simulink model "dynamic_bicycle"  (R2019a)
settings: Solver=VariableStepAuto  StartTime=0.0  StopTime=20  RelTol=1e-3
values from neighbouring files (symbols this model uses):
  cornering_stiffness_front = 10000    [config_dynamic_bicycle.m]
  cornering_stiffness_rear = 10000    [config_dynamic_bicycle.m]
  init_states = [0,0,0,0,0,0]    [config_dynamic_bicycle.m]
  length_front = 1    [config_dynamic_bicycle.m]
  length_rear = 1    [config_dynamic_bicycle.m]
  mass = 200    [config_dynamic_bicycle.m]
  yaw_inertia = 50    [config_dynamic_bicycle.m]
libraries: simulink x2, simulink_extras x1
settings Model: Creator=jacoboffersen  LastModifiedBy=jacoboffersen

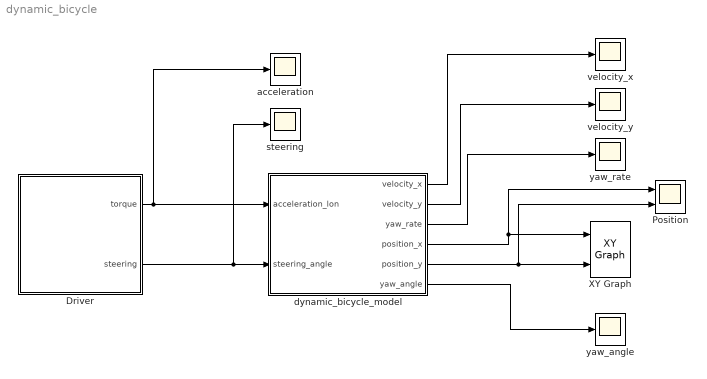
== system dynamic_bicycle ==
  Driver : Subsystem
  Position : Scope  NumInputPorts=2
  XY Graph : simulink/Sinks/XY Graph  xmin=-200  xmax=200  ymin=-200  ymax=200  st=-1
  acceleration : Scope
  "dynamic_bicycle_model " : Subsystem
  steering : Scope
  velocity_x : Scope
  velocity_y : Scope
  yaw_angle : Scope
  yaw_rate : Scope
  wires:
  Driver/2(steering) -> steering/1, "dynamic_bicycle_model "/2(steering_angle)
  Driver/1(torque) -> acceleration/1, "dynamic_bicycle_model "/1(acceleration_lon)
  "dynamic_bicycle_model "/4(position_x) -> Position/1, XY Graph/1
  "dynamic_bicycle_model "/5(position_y) -> Position/2, XY Graph/2
  "dynamic_bicycle_model "/6(yaw_angle) -> yaw_angle/1
  "dynamic_bicycle_model "/3(yaw_rate) -> yaw_rate/1
  "dynamic_bicycle_model "/2(velocity_y) -> velocity_y/1
  "dynamic_bicycle_model "/1(velocity_x) -> velocity_x/1

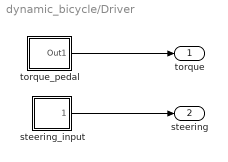
== system dynamic_bicycle/Driver ==
  steering_input : Subsystem
  torque_pedal : Subsystem
  torque : Outport
  steering : Outport  Port=2
  wires:
  torque_pedal/1(Out1) -> torque/1
  steering_input/1(Out1) -> steering/1

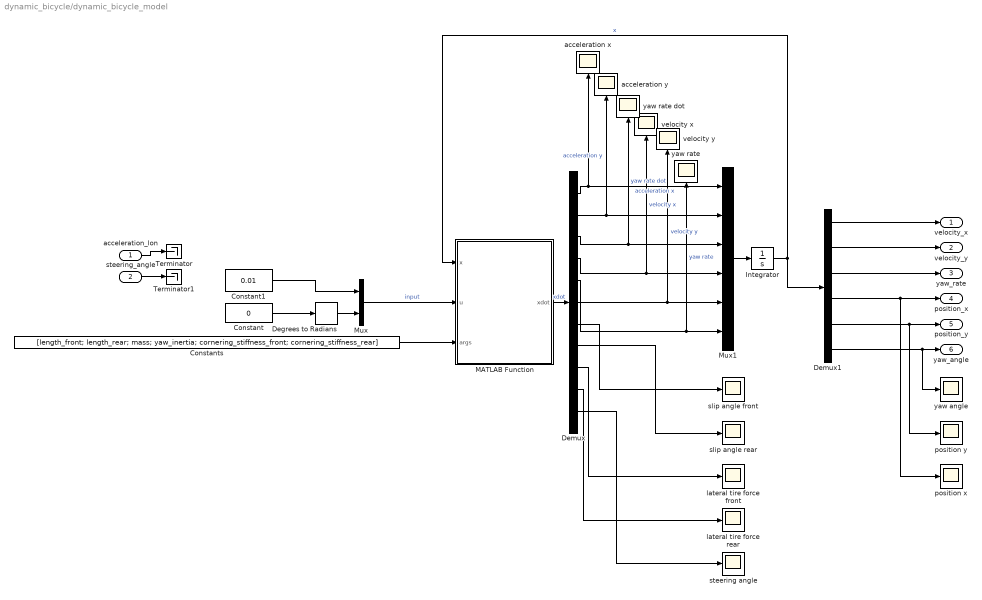
== system dynamic_bicycle/dynamic_bicycle_model  ==
  acceleration_lon : Inport
  steering_angle : Inport  Port=2
  Constant : Constant  Value=0
  Constant1 : Constant  Value=0.01
  Constants : Constant  Value=[length_front; length_rear; mass; yaw_inertia; cornering_stiffness_front; cornering_stiffness_rear]
  Degrees to Radians : simulink_extras/Transformations/Degrees to Radians
  Demux : Demux  Outputs=11
  Demux1 : Demux  Outputs=6
  Integrator : Integrator  InitialCondition=init_states
  MATLAB Function : MATLAB Function  TreatAsAtomicUnit=on
  Mux : Mux  Inputs=2
  Mux1 : Mux  Inputs=6
  Terminator : Terminator
  Terminator1 : Terminator
  acceleration x : Scope
  acceleration y : Scope
  lateral tire force front : Scope
  lateral tire force rear : Scope
  position x : Scope
  position y : Scope
  slip angle front : Scope
  slip angle rear : Scope
  steering angle : Scope
  velocity x : Scope
  velocity y : Scope
  yaw angle : Scope
  yaw rate : Scope
  yaw rate dot : Scope
  velocity_x : Outport
  velocity_y : Outport  Port=2
  yaw_rate : Outport  Port=3
  position_x : Outport  Port=4
  position_y : Outport  Port=5
  yaw_angle : Outport  Port=6
  wires:
  Mux/1 -> MATLAB Function/2(u)  "input"
  Constants/1 -> MATLAB Function/3(args)
  Integrator/1 -> Demux1/1, MATLAB Function/1(x)  "x"
  Demux1/2 -> velocity_y/1
  Demux1/1 -> velocity_x/1
  Demux1/3 -> yaw_rate/1
  Demux1/5 -> position y/1, position_y/1
  Demux1/4 -> position x/1, position_x/1
  Demux1/6 -> yaw angle/1, yaw_angle/1
  Mux1/1 -> Integrator/1
  MATLAB Function/1(xdot) -> Demux/1  "xdot"
  Demux/6 -> yaw rate/1, Mux1/6  "yaw rate"
  Demux/5 -> velocity y/1, Mux1/5  "velocity y"
  Demux/4 -> velocity x/1, Mux1/4  "velocity x"
  Demux/3 -> yaw rate dot/1, Mux1/3  "yaw rate dot"
  Demux/2 -> Mux1/2, acceleration y/1  "acceleration y"
  Demux/1 -> Mux1/1, acceleration x/1  "acceleration x"
  Constant1/1 -> Mux/1
  Degrees to Radians/1 -> Mux/2
  Constant/1 -> Degrees to Radians/1
  Demux/7 -> slip angle front/1
  Demux/8 -> slip angle rear/1
  Demux/11 -> steering angle/1
  Demux/9 -> lateral tire force front/1
  Demux/10 -> lateral tire force rear/1
  steering_angle/1 -> Terminator1/1
  acceleration_lon/1 -> Terminator/1

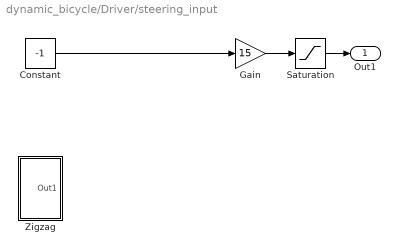
== system dynamic_bicycle/Driver/steering_input ==
  Constant : Constant  Value=-1
  Gain : Gain  Gain=15
  Saturation : Saturate  UpperLimit=30  LowerLimit=-30
  Zigzag : Subsystem
  Out1 : Outport
  wires:
  Saturation/1 -> Out1/1
  Gain/1 -> Saturation/1
  Constant/1 -> Gain/1

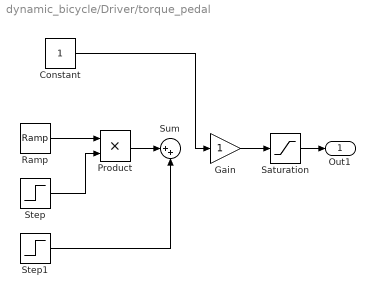
== system dynamic_bicycle/Driver/torque_pedal ==
  Constant : Constant
  Gain : Gain
  Product : Product
  Ramp : simulink/Sources/Ramp  slope=1  start=1  InitialOutput=0
  Saturation : Saturate  UpperLimit=30  LowerLimit=-30
  Step : Step  Time=5  Before=1  After=0  SampleTime=0
  Step1 : Step  Time=5  After=0  SampleTime=0
  Sum : Sum  Inputs=|++
  Out1 : Outport
  wires:
  Saturation/1 -> Out1/1
  Gain/1 -> Saturation/1
  Ramp/1 -> Product/1
  Step/1 -> Product/2
  Product/1 -> Sum/1
  Constant/1 -> Gain/1
  Step1/1 -> Sum/2

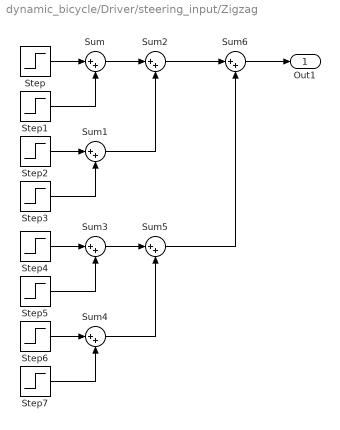
== system dynamic_bicycle/Driver/steering_input/Zigzag ==
  Step : Step  Time=4  SampleTime=0
  Step1 : Step  Time=6  After=-1  SampleTime=0
  Step2 : Step  Time=8  After=-1  SampleTime=0
  Step3 : Step  Time=10  SampleTime=0
  Step4 : Step  Time=12  SampleTime=0
  Step5 : Step  Time=14  After=-1  SampleTime=0
  Step6 : Step  Time=16  After=-1  SampleTime=0
  Step7 : Step  Time=18  SampleTime=0
  Sum{,1..6} (7 alike) : Sum  Inputs=|++
  Out1 : Outport
  wires:
  Step2/1 -> Sum1/1
  Sum5/1 -> Sum6/2
  Sum3/1 -> Sum5/1
  Sum2/1 -> Sum6/1
  Step4/1 -> Sum3/1
  Sum1/1 -> Sum2/2
  Step3/1 -> Sum1/2
  Step/1 -> Sum/1
  Step5/1 -> Sum3/2
  Sum/1 -> Sum2/1
  Step7/1 -> Sum4/2
  Step6/1 -> Sum4/1
  Sum6/1 -> Out1/1
  Sum4/1 -> Sum5/2
  Step1/1 -> Sum/2

== matlab function dynamic_bicycle/dynamic_bicycle_model /MATLAB Function ==
  data: x input; xdot output; u input; args input
function xdot = fcn(x, u, args)

velocity_x = x(1); % x velocity
velocity_y = x(2); % y velocity
yaw_rate   = x(3); % Yaw rate
position_x = x(4);
position_y = x(5);
yaw_angle  = x(6);

acceleation_x   = u(1); % 
steering_angle  = u(2); % Steering angle

length_front              = args(1); % Length from front axle to CG
length_rear               = args(2); % Length from rear  axle to CG
mass                      = args(3);
yaw_inertia               = args(4);
cornering_stiffness_front = args(5);
cornering_stiffness_rear  = args(6);


% ********* Default *********
slip_angle_front    = 0;
slip_angle_rear     = 0;

% 
% slip_angle_front = steering_angle*0.1 * (velocity_x);
% slip_angle_rear  = steering_angle*0.01 * (velocity_x);
% slip_angle_front = steering_angle - (length_front*yaw_rate + velocity_y)/velocity_x;
if(velocity_x > 0.001 || velocity_x < -0.001)
    slip_angle_front = steering_angle - (yaw_rate + velocity_y)/velocity_x;
    slip_angle_front = max(min(slip_angle_front, 10),-10);
  
    
    % slip_angle_rear = (length_rear*yaw_rate+velocity_y)/velocity_x;
    slip_angle_rear = (yaw_rate+velocity_y)/velocity_x;
    slip_angle_rear = max(min(slip_angle_rear, 10), -10);
end




% lat_tire_force_front = -cornering_stiffness_front * slip_angle_front; 
lat_tire_force_front = cornering_stiffness_front * slip_angle_front; 
% lat_tire_force_front = -100 * steering_angle * 0.1;

% lat_tire_force_rear  = -cornering_stiffness_rear  * slip_angle_rear;
lat_tire_force_rear  = cornering_stiffness_rear  * slip_angle_rear;
% lat_tire_force_rear  = -100 * steering_angle * 0.05; 

% acceleration_x_cg   = yaw_rate * velocity_y + acceleation_x;
acceleration_x_cg   = acceleation_x + yaw_rate * velocity_y;


% acceleration_y_cg   = -yaw_rate * velocity_x + (2 * (lat_tire_force_front * cos(steering_angle) + lat_tire_force_rear))/mass;
acceleration_y_cg   = (2 * (lat_tire_force_front * cos(steering_angle) + lat_tire_force_rear))/mass - yaw_rate * velocity_x;

% yaw_rate_dot        = (2 * (length_front * lat_tire_force_front - length_rear * lat_tire_force_rear))/yaw_inertia;
yaw_rate_dot        = (2 * (lat_tire_force_front - lat_tire_force_rear))/yaw_inertia;

% velocity_x_cg       = velocity_x * cos(yaw_angle) - velocity_y * sin(yaw_angle);
velocity_x_cg       = velocity_x * cos(yaw_angle) - velocity_y * sin(yaw_angle);

% velocity_y_cg       = velocity_x * sin(yaw_angle) - velocity_y * cos(yaw_angle);
velocity_y_cg       = velocity_x * sin(yaw_angle) - velocity_y * cos(yaw_angle);
% velocity_y_cg       = velocity_x * sin(yaw_angle) + velocity_y * cos(yaw_angle);




xdot = [acceleration_x_cg; 
        acceleration_y_cg; 
        yaw_rate_dot; 
        velocity_x_cg; 
        velocity_y_cg; 
        yaw_rate; 
        slip_angle_front; 
        slip_angle_rear; 
        lat_tire_force_front;
        lat_tire_force_rear;
        steering_angle];
